simulink model "Final_project_template"  (R2020a)
settings: Solver=FixedStepDiscrete  StartTime=0.0  StopTime=10.0  FixedStep=0.0005  RelTol=1e-3  EnableMultiTasking=on
InitFcn:
  | mbd_s32k_consistency_checks(bdroot(gcs));
values from neighbouring files (symbols this model uses):
  b = 100    [parameters_template.m]
  base_ids = [10, 20, 30, 40, 50, 60]    [parameters_template.m]
  dT = 0.01    [parameters_template.m]
  H = 20    [parameters_template.m]
  L1 = 1.6    [parameters_template.m]
  L2 = 0.8    [parameters_template.m]
  m = 2000    [parameters_template.m]
  n_desired = 0    [parameters_template.m]
  pot_gain = 1    [parameters_template.m]
  pot_offset = 512    [parameters_template.m]
  R = 1/5    (= 0.2)    [parameters_template.m]
  S_Kd1 = 0.05    [parameters_template.m]
  S_Kd2 = 100    [parameters_template.m]
  S_Kp1 = 0.5    [parameters_template.m]
  S_Kp2 = 1000    [parameters_template.m]
  V_Ki = 50    [parameters_template.m]
  V_Kp = 5000    [parameters_template.m]
undefined symbols (not defined in the file or in its folder): A, DiscIntNeverNeededParam, LQFP
libraries: mbd_s32k1xx_ec_toolbox x38, xpcutilitieslib x15, Veh_Sim x9, simulink x3
(part 2 of 2)

== system Final_project_template/High Level Design/Outputs/Tx CAN ==
  note: Use pack block to generate data arrays
      | Do not use any mailbox buffers that are used for receives
  note: Use FCAN_Send block to transmit two messages to the CAN bus
  s,n,psi,us : Inport
  "Byte Packing " : xpcutilitieslib/Byte Packing   MaskPackedDataType=uint8  MaskUnpackedDataTypes={'single'}  MaskAlignment=1
  Byte Packing 1 : xpcutilitieslib/Byte Packing   MaskPackedDataType=uint8  MaskUnpackedDataTypes={'single'}  MaskAlignment=1
  Constant : Constant  Value=8  OutDataTypeStr=uint8
  Constant2 : Constant  Value=8  OutDataTypeStr=uint8
  Demux : Demux  Outputs=2
  FCAN_Send : mbd_s32k1xx_ec_toolbox/Communication Blocks/CAN Blocks/FCAN_Send  can_instance=0  can_mode=Non-blocking  can_timeout_ms=0  can_mb_idx=0  can_extended_id=off  can_is_remote=off  can_id=19  show_adv_opts=on  can_fd_enable=off  can_enable_brs=off  can_fd_padding=0
  FCAN_Send1 : mbd_s32k1xx_ec_toolbox/Communication Blocks/CAN Blocks/FCAN_Send  can_instance=0  can_mode=Non-blocking  can_timeout_ms=0  can_mb_idx=1  can_extended_id=off  can_is_remote=off  can_id=1A  show_adv_opts=off  can_fd_enable=off  can_enable_brs=off  can_fd_padding=0
  wires:
  s,n,psi,us/1 -> Demux/1
  Demux/1 -> "Byte Packing "/1
  Demux/2 -> Byte Packing 1/1
  "Byte Packing "/1 -> FCAN_Send/1
  Byte Packing 1/1 -> FCAN_Send1/1
  Constant/1 -> FCAN_Send/2
  Constant2/1 -> FCAN_Send1/2

== system Final_project_template/High Level Design/Outputs/write torque ==
  Reaction Torque : Inport
  Constant : Constant  Value=0  OutDataTypeStr=single
  Data Type Conversion : DataTypeConversion  OutDataTypeStr=single
  FTM_PWM_Config : mbd_s32k1xx_ec_toolbox/Motor Control Blocks/FTM Blocks/FTM_PWM_Config  ftmModule=0  ftmMode=Edge-Aligned PWM  ftmSourceClock=80 MHz  swcontrol_enable=off  chan0En=on  chan0Type=Independent  chan2En=off  chan2Type=Independent  chan4En=off  chan4Type=Independent  chan6En=off  chan6Type=Independent  ftmPwmUnits=Hz  outFrequency=20000  ftmPeriod=4000  ftmPrescaler=Divide by 1  deadtimeUnits=Nanoseconds  deadtimeNs=0  deadtimeTicks=0  deadtimePrescaler=Divide by 1  dutyCycleCh0=0.5  dutyCycleCh1=0.25  dutyCycleCh2=0.25  dutyCycleCh3=0.25  dutyCycleCh4=0.25  dutyCycleCh5=0.25  dutyCycleCh6=0.25  dutyCycleCh7=0.25  dutyCycleSim=on  startAfterInit=on  showAdvOpt=on  pinFtmCh0=PTB12: [FTM0_CH0 | FTM Channel]  pinFtmCh1=None  pinPolCh0=Active High  pinPolCh1=Active Low  outputComplem0=Main duplicated  outputLevel0=Low  outputLevel1=Low  pinFtmCh2=PTC2: [FTM0_CH2 | FTM Channel]  pinFtmCh3=None  pinPolCh2=Active Low  pinPolCh3=Active Low  outputComplem2=Main duplicated  outputLevel2=Low  outputLevel3=Low  pinFtmCh4=PTB4: [FTM0_CH4 | FTM Channel]  pinFtmCh5=None  pinPolCh4=Active Low  pinPolCh5=Active Low  outputComplem4=Main duplicated  outputLevel4=Low  outputLevel5=Low  pinFtmCh6=PTA17: [FTM0_CH6 | FTM Channel]  pinFtmCh7=None  pinPolCh6=Active Low  pinPolCh7=Active Low  outputComplem6=Main duplicated  outputLevel6=Low  outputLevel7=Low  initTrigger=off  chTrigger0=off  chTrigger1=off  chTrigger2=off  chTrigger3=off  chTrigger4=off  chTrigger5=off  chTrigger6=off  chTrigger7=off  mcuTargetUpdate=on  pwmSyncTrg=Software trigger  pwmSyncHwRouting=TRGMUX_FTM7  pwmSyncTrg0=off  pwmSyncTrg1=off  pwmSyncTrg2=off  pwmSyncAutoClear=on  pwmSyncMinLoad=on  pwmSyncMaxLoad=on  pwmSyncInvert=System Clock  pwmSyncOutControl=System Clock  pwmSyncOutMask=System Clock  pwmSyncCounterInitial=System Clock  pwmSyncPoints=Update now  reloadEnable=off  reloadPriority=15  reloadHalfCycle=off  reloadHCR=0  reloadFrequency=0  chnMatch0=off  chnMatch1=off  chnMatch2=off  chnMatch3=off  chnMatch4=off  chnMatch5=off  chnMatch6=off  chnMatch7=off  pwmFaultProtection=off  pwmFaultInterrupt=off  pwmFaultClearing=Fault control disabled  pwmFaultPinState=Safe Value  pwmFaultFilterValue=0  pwmFaultPriority=15  fault_disen_0=off  fault_filter_0=off  fault_polarity_0=Active High  fault_disen_1=off  fault_filter_1=off  fault_polarity_1=Active high  fault_disen_2=off  fault_filter_2=off  fault_polarity_2=Active high  fault_disen_3=off  fault_filter_3=off  fault_polarity_3=Active high  fault_pin_0=None  fault_pin_1=None  fault_pin_2=None  fault_pin_3=None
  Subsystem1 : Subsystem
  Terminator1 : Terminator
  Terminator3 : Terminator
  wires:
  Reaction Torque/1 -> Subsystem1/1(torque)
  Subsystem1/1(dutycycle) -> Data Type Conversion/1
  Data Type Conversion/1 -> FTM_PWM_Config/1
  Constant/1 -> FTM_PWM_Config/2
  FTM_PWM_Config/2 -> Terminator1/1
  FTM_PWM_Config/1 -> Terminator3/1

== system Final_project_template/High Level Design/Vehicle Dynamics/Subsystem ==
  u : Inport
  delta : Inport  Port=2
  Gain : Gain  Gain=-A
  Product : Product
  Self-Aligning Torque : Outport
  wires:
  Product/1 -> Gain/1
  u/1 -> Product/1
  delta/1 -> Product/2
  Gain/1 -> Self-Aligning Torque/1

== system Final_project_template/Serial Sim Out to Virtual Sim/UART Iteration/Resettable Subsystem ==
  Reset : ResetPort  DisableCoverage=on  ResetTriggerType=either
  Constant : Constant
  Delay : Delay  DelayLength=1
  Sum : Sum  Inputs=|++
  Out1 : Outport  VectorParamsAs1DForOutWhenUnconnected=off
  wires:
  Delay/1 -> Sum/1
  Constant/1 -> Sum/2
  Sum/1 -> Out1/1, Delay/1

== system Final_project_template/Can Network Inputs/Extract CAN data/Data to s,n,psi,us /Switch Case Action Subsystem2 ==
  s,n : Inport
  Action Port : ActionPort  ActionPortLabel=if(u1 == 5)
  "Byte Unpacking " : xpcutilitieslib/Byte Unpacking   MaskUnpackedDataTypes={'single', 'single'}  MaskUnpackedDataSizes={[1], [1]}  MaskAlignment=1
      settings: SourceProductBaseCode=XP
  s : Outport  VectorParamsAs1DForOutWhenUnconnected=off
  n : Outport  Port=2  VectorParamsAs1DForOutWhenUnconnected=off
  wires:
  s,n/1 -> "Byte Unpacking "/1
  "Byte Unpacking "/1 -> s/1
  "Byte Unpacking "/2 -> n/1

== system Final_project_template/Can Network Inputs/Extract CAN data/Data to s,n,psi,us /Switch Case Action Subsystem3 ==
  psi,us : Inport
  Action Port : ActionPort  ActionPortLabel=elseif(u1 == 6)
  "Byte Unpacking " : xpcutilitieslib/Byte Unpacking   MaskUnpackedDataTypes={'single', 'single'}  MaskUnpackedDataSizes={[1], [1]}  MaskAlignment=1
      settings: SourceProductBaseCode=XP
  psi : Outport  VectorParamsAs1DForOutWhenUnconnected=off
  us : Outport  Port=2  VectorParamsAs1DForOutWhenUnconnected=off
  wires:
  psi,us/1 -> "Byte Unpacking "/1
  "Byte Unpacking "/1 -> psi/1
  "Byte Unpacking "/2 -> us/1

== system Final_project_template/Can Network Inputs/Extract CAN data/Data to s,n,psi,us 1/Switch Case Action Subsystem2 ==
  s,n : Inport
  Action Port : ActionPort  ActionPortLabel=if(u1 == 5)
  "Byte Unpacking " : xpcutilitieslib/Byte Unpacking   MaskUnpackedDataTypes={'single', 'single'}  MaskUnpackedDataSizes={[1], [1]}  MaskAlignment=1
      settings: SourceProductBaseCode=XP
  s : Outport  VectorParamsAs1DForOutWhenUnconnected=off
  n : Outport  Port=2  VectorParamsAs1DForOutWhenUnconnected=off
  wires:
  s,n/1 -> "Byte Unpacking "/1
  "Byte Unpacking "/1 -> s/1
  "Byte Unpacking "/2 -> n/1

== system Final_project_template/Can Network Inputs/Extract CAN data/Data to s,n,psi,us 1/Switch Case Action Subsystem3 ==
  psi,us : Inport
  Action Port : ActionPort  ActionPortLabel=elseif(u1 == 6)
  "Byte Unpacking " : xpcutilitieslib/Byte Unpacking   MaskUnpackedDataTypes={'single', 'single'}  MaskUnpackedDataSizes={[1], [1]}  MaskAlignment=1
      settings: SourceProductBaseCode=XP
  psi : Outport  VectorParamsAs1DForOutWhenUnconnected=off
  us : Outport  Port=2  VectorParamsAs1DForOutWhenUnconnected=off
  wires:
  psi,us/1 -> "Byte Unpacking "/1
  "Byte Unpacking "/1 -> psi/1
  "Byte Unpacking "/2 -> us/1

== system Final_project_template/Can Network Inputs/Extract CAN data/Data to s,n,psi,us 2/Switch Case Action Subsystem2 ==
  s,n : Inport
  Action Port : ActionPort  ActionPortLabel=if(u1 == 5)
  "Byte Unpacking " : xpcutilitieslib/Byte Unpacking   MaskUnpackedDataTypes={'single', 'single'}  MaskUnpackedDataSizes={[1], [1]}  MaskAlignment=1
      settings: SourceProductBaseCode=XP
  s : Outport  VectorParamsAs1DForOutWhenUnconnected=off
  n : Outport  Port=2  VectorParamsAs1DForOutWhenUnconnected=off
  wires:
  s,n/1 -> "Byte Unpacking "/1
  "Byte Unpacking "/1 -> s/1
  "Byte Unpacking "/2 -> n/1

== system Final_project_template/Can Network Inputs/Extract CAN data/Data to s,n,psi,us 2/Switch Case Action Subsystem3 ==
  psi,us : Inport
  Action Port : ActionPort  ActionPortLabel=elseif(u1 == 6)
  "Byte Unpacking " : xpcutilitieslib/Byte Unpacking   MaskUnpackedDataTypes={'single', 'single'}  MaskUnpackedDataSizes={[1], [1]}  MaskAlignment=1
      settings: SourceProductBaseCode=XP
  psi : Outport  VectorParamsAs1DForOutWhenUnconnected=off
  us : Outport  Port=2  VectorParamsAs1DForOutWhenUnconnected=off
  wires:
  psi,us/1 -> "Byte Unpacking "/1
  "Byte Unpacking "/1 -> psi/1
  "Byte Unpacking "/2 -> us/1

== system Final_project_template/Can Network Inputs/Extract CAN data/Data to s,n,psi,us 3/Switch Case Action Subsystem2 ==
  s,n : Inport
  Action Port : ActionPort  ActionPortLabel=if(u1 == 5)
  "Byte Unpacking " : xpcutilitieslib/Byte Unpacking   MaskUnpackedDataTypes={'single', 'single'}  MaskUnpackedDataSizes={[1], [1]}  MaskAlignment=1
      settings: SourceProductBaseCode=XP
  s : Outport  VectorParamsAs1DForOutWhenUnconnected=off
  n : Outport  Port=2  VectorParamsAs1DForOutWhenUnconnected=off
  wires:
  s,n/1 -> "Byte Unpacking "/1
  "Byte Unpacking "/1 -> s/1
  "Byte Unpacking "/2 -> n/1

== system Final_project_template/Can Network Inputs/Extract CAN data/Data to s,n,psi,us 3/Switch Case Action Subsystem3 ==
  psi,us : Inport
  Action Port : ActionPort  ActionPortLabel=elseif(u1 == 6)
  "Byte Unpacking " : xpcutilitieslib/Byte Unpacking   MaskUnpackedDataTypes={'single', 'single'}  MaskUnpackedDataSizes={[1], [1]}  MaskAlignment=1
      settings: SourceProductBaseCode=XP
  psi : Outport  VectorParamsAs1DForOutWhenUnconnected=off
  us : Outport  Port=2  VectorParamsAs1DForOutWhenUnconnected=off
  wires:
  psi,us/1 -> "Byte Unpacking "/1
  "Byte Unpacking "/1 -> psi/1
  "Byte Unpacking "/2 -> us/1

== system Final_project_template/Can Network Inputs/Extract CAN data/Data to s,n,psi,us 4/Switch Case Action Subsystem2 ==
  s,n : Inport
  Action Port : ActionPort  ActionPortLabel=if(u1 == 5)
  "Byte Unpacking " : xpcutilitieslib/Byte Unpacking   MaskUnpackedDataTypes={'single', 'single'}  MaskUnpackedDataSizes={[1], [1]}  MaskAlignment=1
      settings: SourceProductBaseCode=XP
  s : Outport  VectorParamsAs1DForOutWhenUnconnected=off
  n : Outport  Port=2  VectorParamsAs1DForOutWhenUnconnected=off
  wires:
  s,n/1 -> "Byte Unpacking "/1
  "Byte Unpacking "/1 -> s/1
  "Byte Unpacking "/2 -> n/1

== system Final_project_template/Can Network Inputs/Extract CAN data/Data to s,n,psi,us 4/Switch Case Action Subsystem3 ==
  psi,us : Inport
  Action Port : ActionPort  ActionPortLabel=elseif(u1 == 6)
  "Byte Unpacking " : xpcutilitieslib/Byte Unpacking   MaskUnpackedDataTypes={'single', 'single'}  MaskUnpackedDataSizes={[1], [1]}  MaskAlignment=1
      settings: SourceProductBaseCode=XP
  psi : Outport  VectorParamsAs1DForOutWhenUnconnected=off
  us : Outport  Port=2  VectorParamsAs1DForOutWhenUnconnected=off
  wires:
  psi,us/1 -> "Byte Unpacking "/1
  "Byte Unpacking "/1 -> psi/1
  "Byte Unpacking "/2 -> us/1

== system Final_project_template/Can Network Inputs/Extract CAN data/Data to s,n,psi,us 5/Switch Case Action Subsystem2 ==
  s,n : Inport
  Action Port : ActionPort  ActionPortLabel=if(u1 == 5)
  "Byte Unpacking " : xpcutilitieslib/Byte Unpacking   MaskUnpackedDataTypes={'single', 'single'}  MaskUnpackedDataSizes={[1], [1]}  MaskAlignment=1
      settings: SourceProductBaseCode=XP
  s : Outport  VectorParamsAs1DForOutWhenUnconnected=off
  n : Outport  Port=2  VectorParamsAs1DForOutWhenUnconnected=off
  wires:
  s,n/1 -> "Byte Unpacking "/1
  "Byte Unpacking "/1 -> s/1
  "Byte Unpacking "/2 -> n/1

== system Final_project_template/Can Network Inputs/Extract CAN data/Data to s,n,psi,us 5/Switch Case Action Subsystem3 ==
  psi,us : Inport
  Action Port : ActionPort  ActionPortLabel=elseif(u1 == 6)
  "Byte Unpacking " : xpcutilitieslib/Byte Unpacking   MaskUnpackedDataTypes={'single', 'single'}  MaskUnpackedDataSizes={[1], [1]}  MaskAlignment=1
      settings: SourceProductBaseCode=XP
  psi : Outport  VectorParamsAs1DForOutWhenUnconnected=off
  us : Outport  Port=2  VectorParamsAs1DForOutWhenUnconnected=off
  wires:
  psi,us/1 -> "Byte Unpacking "/1
  "Byte Unpacking "/1 -> psi/1
  "Byte Unpacking "/2 -> us/1

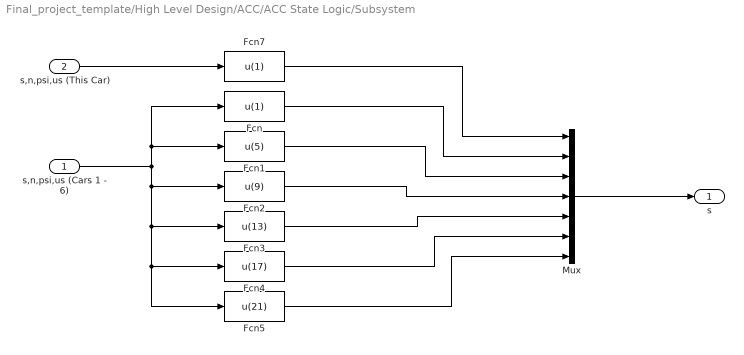
== system Final_project_template/High Level Design/ACC/ACC State Logic/Subsystem ==
  s,n,psi,us (Cars 1 - 6) : Inport
  s,n,psi,us (This Car) : Inport  Port=2
  Fcn : Fcn  Expr=u(1)
  Fcn1 : Fcn  Expr=u(5)
  Fcn2 : Fcn  Expr=u(9)
  Fcn3 : Fcn  Expr=u(13)
  Fcn4 : Fcn  Expr=u(17)
  Fcn5 : Fcn  Expr=u(21)
  Fcn7 : Fcn  Expr=u(1)
  Mux : Mux  Inputs=7
  s : Outport
  wires:
  Mux/1 -> s/1
  s,n,psi,us (This Car)/1 -> Fcn7/1
  s,n,psi,us (Cars 1 - 6)/1 -> Fcn5/1, Fcn4/1, Fcn3/1, Fcn2/1, Fcn1/1, Fcn/1
  Fcn7/1 -> Mux/1
  Fcn/1 -> Mux/2
  Fcn1/1 -> Mux/3
  Fcn2/1 -> Mux/4
  Fcn3/1 -> Mux/5
  Fcn4/1 -> Mux/6
  Fcn5/1 -> Mux/7

== system Final_project_template/High Level Design/ACC/ACC State Logic/Subsystem2 ==
  s,n,psi,us (Cars 1 - 6) : Inport
  s,n,psi,us (This Car) : Inport  Port=2
  Fcn : Fcn  Expr=u(4)
  Fcn1 : Fcn  Expr=u(8)
  Fcn2 : Fcn  Expr=u(12)
  Fcn3 : Fcn  Expr=u(16)
  Fcn4 : Fcn  Expr=u(20)
  Fcn5 : Fcn  Expr=u(24)
  Fcn7 : Fcn  Expr=u(4)
  Mux : Mux  Inputs=7
  u : Outport
  wires:
  Mux/1 -> u/1
  s,n,psi,us (This Car)/1 -> Fcn7/1
  s,n,psi,us (Cars 1 - 6)/1 -> Fcn5/1, Fcn4/1, Fcn3/1, Fcn2/1, Fcn1/1, Fcn/1
  Fcn7/1 -> Mux/1
  Fcn/1 -> Mux/2
  Fcn1/1 -> Mux/3
  Fcn2/1 -> Mux/4
  Fcn3/1 -> Mux/5
  Fcn4/1 -> Mux/6
  Fcn5/1 -> Mux/7

== system Final_project_template/High Level Design/ACC/Speed Ctrl/PI ==
  Error : Inport
  Gain : Gain  Gain=V_Ki  SaturateOnIntegerOverflow=on  OutDataTypeStr=Inherit: Same as input  ParamDataTypeStr=Inherit: Same as input
  Gain1 : Gain  Gain=V_Kp  SaturateOnIntegerOverflow=on  OutDataTypeStr=Inherit: Same as input  ParamDataTypeStr=Inherit: Same as input
  My Discrete Integrator : Subsystem
  Sum : Sum  Inputs=|++  SaturateOnIntegerOverflow=on
  U : Outport
  wires:
  Sum/1 -> U/1
  Error/1 -> Gain1/1, Gain/1
  Gain1/1 -> Sum/2
  My Discrete Integrator/1(X) -> Sum/1
  Gain/1 -> My Discrete Integrator/1(X_dot)

== system Final_project_template/High Level Design/Inputs/get wheel position/Subsystem ==
  encoder count : Inport
  Data Type Conversion : DataTypeConversion  OutDataTypeStr=uint16
  Data Type Conversion1 : DataTypeConversion  OutDataTypeStr=int16
  Data Type Conversion2 : DataTypeConversion  OutDataTypeStr=single
  Delay : Delay  DelayLength=1  InitialCondition=0
  Delay1 : Delay  DelayLength=1  InitialCondition=0
  Gain : Gain  Gain=0.09
  Gain1 : Gain  Gain=-3.14159264/180
  Sum : Sum  Inputs=|++
  Sum1 : Sum  Inputs=|+-
  radians : Outport
  wires:
  Data Type Conversion1/1 -> Data Type Conversion2/1
  encoder count/1 -> Data Type Conversion/1
  Data Type Conversion2/1 -> Gain/1
  Data Type Conversion/1 -> Delay/1, Sum1/1
  Delay/1 -> Sum1/2
  Sum1/1 -> Data Type Conversion1/1
  Gain/1 -> Sum/1
  Delay1/1 -> Sum/2
  Sum/1 -> Delay1/1, Gain1/1
  Gain1/1 -> radians/1

== system Final_project_template/High Level Design/Outputs/Extract x,y,psi (Cars 1 - 6)/Extract x,y,psi ==
  s,n,psi,us : Inport
  Demux : Demux
  Mux : Mux  Inputs=3
  Terminator : Terminator
  s,n to x,y : Veh_Sim/s,n to x,y  SystemSampleTime=-1  Latency=0  AutoFrameSizeCalculation=off
  x,y,psi : Outport  VectorParamsAs1DForOutWhenUnconnected=off
  wires:
  Demux/1 -> s,n to x,y/1
  Demux/2 -> s,n to x,y/2
  s,n,psi,us/1 -> Demux/1
  s,n to x,y/1 -> Mux/1
  s,n to x,y/2 -> Mux/2
  Demux/3 -> Mux/3
  Mux/1 -> x,y,psi/1
  Demux/4 -> Terminator/1

== system Final_project_template/High Level Design/Outputs/Extract x,y,psi (Cars 1 - 6)/Extract x,y,psi1 ==
  s,n,psi,us : Inport
  Demux : Demux
  Mux : Mux  Inputs=3
  Terminator : Terminator
  s,n to x,y : Veh_Sim/s,n to x,y  SystemSampleTime=-1  Latency=0  AutoFrameSizeCalculation=off
  x,y,psi : Outport  VectorParamsAs1DForOutWhenUnconnected=off
  wires:
  Demux/1 -> s,n to x,y/1
  Demux/2 -> s,n to x,y/2
  s,n,psi,us/1 -> Demux/1
  s,n to x,y/1 -> Mux/1
  s,n to x,y/2 -> Mux/2
  Demux/3 -> Mux/3
  Mux/1 -> x,y,psi/1
  Demux/4 -> Terminator/1

== system Final_project_template/High Level Design/Outputs/Extract x,y,psi (Cars 1 - 6)/Extract x,y,psi2 ==
  s,n,psi,us : Inport
  Demux : Demux
  Mux : Mux  Inputs=3
  Terminator : Terminator
  s,n to x,y : Veh_Sim/s,n to x,y  SystemSampleTime=-1  Latency=0  AutoFrameSizeCalculation=off
  x,y,psi : Outport  VectorParamsAs1DForOutWhenUnconnected=off
  wires:
  Demux/1 -> s,n to x,y/1
  Demux/2 -> s,n to x,y/2
  s,n,psi,us/1 -> Demux/1
  s,n to x,y/1 -> Mux/1
  s,n to x,y/2 -> Mux/2
  Demux/3 -> Mux/3
  Mux/1 -> x,y,psi/1
  Demux/4 -> Terminator/1

== system Final_project_template/High Level Design/Outputs/Extract x,y,psi (Cars 1 - 6)/Extract x,y,psi3 ==
  s,n,psi,us : Inport
  Demux : Demux
  Mux : Mux  Inputs=3
  Terminator : Terminator
  s,n to x,y : Veh_Sim/s,n to x,y  SystemSampleTime=-1  Latency=0  AutoFrameSizeCalculation=off
  x,y,psi : Outport  VectorParamsAs1DForOutWhenUnconnected=off
  wires:
  Demux/1 -> s,n to x,y/1
  Demux/2 -> s,n to x,y/2
  s,n,psi,us/1 -> Demux/1
  s,n to x,y/1 -> Mux/1
  s,n to x,y/2 -> Mux/2
  Demux/3 -> Mux/3
  Mux/1 -> x,y,psi/1
  Demux/4 -> Terminator/1

== system Final_project_template/High Level Design/Outputs/Extract x,y,psi (Cars 1 - 6)/Extract x,y,psi4 ==
  s,n,psi,us : Inport
  Demux : Demux
  Mux : Mux  Inputs=3
  Terminator : Terminator
  s,n to x,y : Veh_Sim/s,n to x,y  SystemSampleTime=-1  Latency=0  AutoFrameSizeCalculation=off
  x,y,psi : Outport  VectorParamsAs1DForOutWhenUnconnected=off
  wires:
  Demux/1 -> s,n to x,y/1
  Demux/2 -> s,n to x,y/2
  s,n,psi,us/1 -> Demux/1
  s,n to x,y/1 -> Mux/1
  s,n to x,y/2 -> Mux/2
  Demux/3 -> Mux/3
  Mux/1 -> x,y,psi/1
  Demux/4 -> Terminator/1

== system Final_project_template/High Level Design/Outputs/Extract x,y,psi (Cars 1 - 6)/Extract x,y,psi5 ==
  s,n,psi,us : Inport
  Demux : Demux
  Mux : Mux  Inputs=3
  Terminator : Terminator
  s,n to x,y : Veh_Sim/s,n to x,y  SystemSampleTime=-1  Latency=0  AutoFrameSizeCalculation=off
  x,y,psi : Outport  VectorParamsAs1DForOutWhenUnconnected=off
  wires:
  Demux/1 -> s,n to x,y/1
  Demux/2 -> s,n to x,y/2
  s,n,psi,us/1 -> Demux/1
  s,n to x,y/1 -> Mux/1
  s,n to x,y/2 -> Mux/2
  Demux/3 -> Mux/3
  Mux/1 -> x,y,psi/1
  Demux/4 -> Terminator/1

== system Final_project_template/High Level Design/Outputs/write torque/Subsystem1 ==
  torque : Inport
  Constant : Constant  Value=0.5  OutDataTypeStr=single
  Gain : Gain  Gain=0.0003162
  Saturation : Saturate  UpperLimit=0.76  LowerLimit=0.24
  Sum : Sum  Inputs=|++
  dutycycle : Outport
  wires:
  Constant/1 -> Sum/2
  Gain/1 -> Sum/1
  torque/1 -> Gain/1
  Sum/1 -> Saturation/1
  Saturation/1 -> dutycycle/1

== system Final_project_template/High Level Design/ACC/Speed Ctrl/PI/My Discrete Integrator ==
  X_dot : Inport
  Gain : Gain  Gain=dT  SaturateOnIntegerOverflow=on  OutDataTypeStr=Inherit: Same as input  ParamDataTypeStr=Inherit: Same as input
  Sum : Sum  Inputs=|++  InputSameDT=on  SaturateOnIntegerOverflow=on  OutDataTypeStr=Inherit: Same as first input
  Unit Delay : UnitDelay  SampleTime=-1  HasFrameUpgradeWarning=on
  X : Outport
  wires:
  Gain/1 -> Sum/1
  X_dot/1 -> Gain/1
  Sum/1 -> Unit Delay/1
  Unit Delay/1 -> Sum/2, X/1

== stateflow chart Final_project_template/High Level Design/ACC/ACC State Logic/Choose_Mode ==
  state Manual
    entry: en_man=true;
    en_vel = false;
    en_pos = false;
  state Position
    entry: en_man=false;
    en_vel = false;
    en_pos = true;
  state Velocity
    entry: en_man=false ;
    en_vel = true;
    en_pos = false;
  (default) -> Manual
  Manual -> Position [order 1] : [(En_Man==0) & ((Usi<=Us) & (Si-S<=H+1))&(Si~=S)]
  Manual -> Velocity [order 2] : [(En_Man==0) &((Usi>Us) | (Si-S>H+1) | (Si==S))]
  Velocity -> Manual [order 1] : [En_Man==1]
  Position -> Manual [order 2] : [En_Man==1]
  Velocity -> Position [order 2] : [(En_Man==0) & ((Usi<=Us) & (Si-S<=H+1))&(Si~=S)]
  Position -> Velocity [order 1] : [(En_Man==0) &((Usi>Us) | (Si-S>H+1) | (Si==S))]
  data: en_man output boolean; en_vel output boolean; en_pos output boolean; En_Man input boolean; Usi input single; Us input single; H input single; Si input single; S input single
